simulink model "controlled_IPD_from_ISO"  (Simulink 7.9)
settings: Solver=ode45  StartTime=0  StopTime=5  FixedStep=0.001  MinStep=0.0001  RelTol=1e-3
libraries: simulink x1
settings Model: Creator=compiaffe  LastModifiedBy=compiaffe

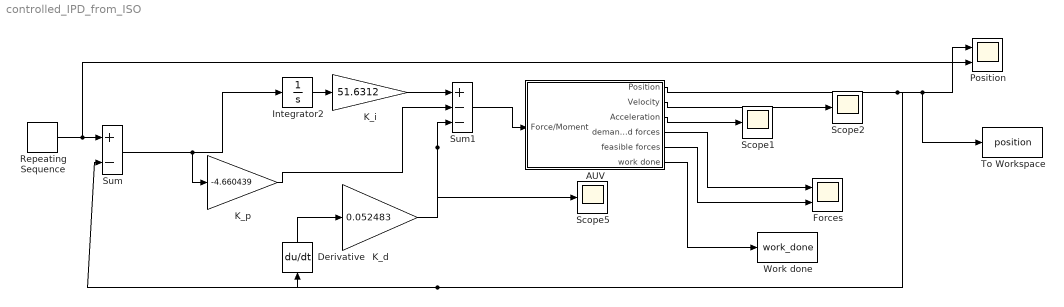
== system controlled_IPD_from_ISO ==
  AUV : Subsystem
  Derivative : Derivative
  Forces : Scope  NumInputPorts=2
      settings: TickLabels=on  ShowLegends=on  YMin=-25~-25  YMax=20~20  SaveName=ScopeData3  MaxDataPoints=500000  SampleTime=1
  Integrator2 : Integrator
  K_d : Gain  Gain=0.052483
  K_i : Gain  Gain=51.6312
  K_p : Gain  Gain=-4.660439
  Position : Scope  NumInputPorts=2
      settings: TickLabels=on  ShowLegends=on  YMin=0~0  YMax=6~5  MaxDataPoints=500000  SampleTime=1
  Repeating Sequence : simulink/Sources/Repeating Sequence  rep_seq_t=[0 1 1 2 2 3 3]  rep_seq_y=[0 0 1 1 5 5 0]
  Scope1 : Scope
      settings: TimeRange=0.16
  Scope2 : Scope
      settings: TimeRange=0.16  SaveName=ScopeData2
  Scope5 : Scope
      settings: TimeRange=0.16  YMin=-10.15  YMax=-9.5  SaveName=ScopeData5
  Sum : Sum  Inputs=+-
  Sum1 : Sum  Inputs=+--
  To Workspace : ToWorkspace  VariableName=position  SampleTime=-1  SaveFormat=Timeseries
  Work done : ToWorkspace  VariableName=work_done  SampleTime=-1  SaveFormat=Timeseries
  wires:
  Repeating Sequence/1 -> Sum/1, Position/2
  Integrator2/1 -> K_i/1
  K_i/1 -> Sum1/1
  Sum1/1 -> AUV/1(Force/Moment)
  AUV/1(Position) -> Position/1, To Workspace/1, Sum/2, Derivative/1
  AUV/2(Velocity) -> Scope2/1
  AUV/3(Acceleration) -> Scope1/1
  K_d/1 -> Scope5/1, Sum1/3
  Derivative/1 -> K_d/1
  K_p/1 -> Sum1/2
  AUV/4(demanded forces) -> Forces/1
  AUV/5(feasible forces) -> Forces/2
  Sum/1 -> Integrator2/1, K_p/1
  AUV/6(work done) -> Work done/1

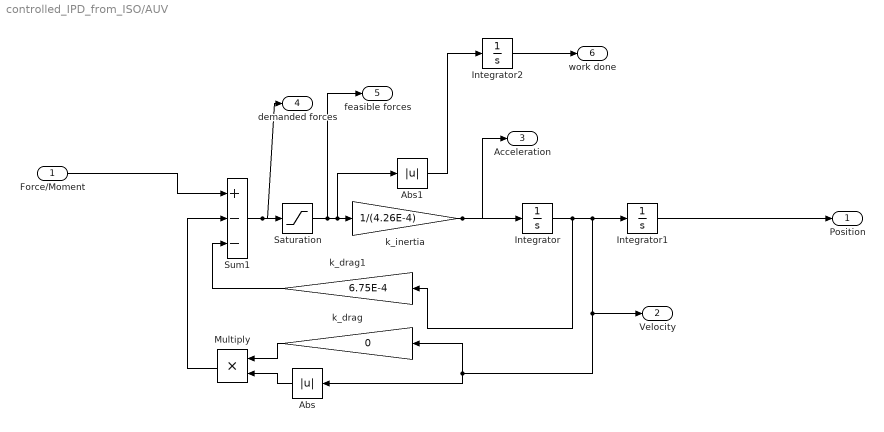
== system controlled_IPD_from_ISO/AUV ==
  Force/Moment : Inport
  Abs : Abs
  Abs1 : Abs
  Integrator : Integrator
  Integrator1 : Integrator
  Integrator2 : Integrator
  Multiply : Product  Inputs=**
  Saturation : Saturate  UpperLimit=28.4  LowerLimit=-28.4
  Sum1 : Sum  Inputs=+--
  k_drag : Gain  Gain=0
  k_drag1 : Gain  Gain=6.75E-4
  k_inertia : Gain  Gain=1/(4.26E-4)
  Position : Outport
  Velocity : Outport  Port=2
  Acceleration : Outport  Port=3
  demanded forces : Outport  Port=4
  feasible forces : Outport  Port=5
  work done : Outport  Port=6
  wires:
  k_drag1/1 -> Sum1/3
  Abs/1 -> Multiply/2
  k_inertia/1 -> Integrator/1, Acceleration/1
  Sum1/1 -> demanded forces/1, Saturation/1
  Multiply/1 -> Sum1/2
  k_drag/1 -> Multiply/1
  Integrator1/1 -> Position/1
  Integrator/1 -> Integrator1/1, Velocity/1, k_drag/1, Abs/1, k_drag1/1
  Force/Moment/1 -> Sum1/1
  Saturation/1 -> feasible forces/1, k_inertia/1, Abs1/1
  Integrator2/1 -> work done/1
  Abs1/1 -> Integrator2/1
